simulink model "CASADI_MPC"  (R2023b)
settings: Solver=FixedStepAuto  StartTime=0.0  StopTime=15  FixedStep=0.002  RelTol=1e-3  EnableMultiTasking=on
undefined symbols (not defined in the file or in its folder): DiscIntNeverNeededParam
settings Model: ExtModeTrigDuration=10000  Creator=franc  LastModifiedBy=franc
settings SolverCC: AlgebraicLoopSolver=TrustRegion  PositivePriorityOrder=on
settings DataIOCC: ReturnWorkspaceOutputs=off
settings OptimizationCC: LifeSpan=inf
settings DebuggingCC: UnconnectedInputMsg=warning  UnconnectedOutputMsg=warning  UnconnectedLineMsg=warning  ArithmeticOperatorsInVariantConditions=warning
settings ModelReferenceCC: EnableRefExpFcnMdlSchedulingChecks=on
settings SFSimCC: SimUseLocalCustomCode=off  CustomCodeUndefinedFunction=UseInterfaceOnly
settings RTWCC: Description=QUARC Win64 Target  SystemTargetFile=quarc_win64.tlc  TemplateMakefile=quarc_default_tmf  RTWUseLocalCustomCode=off
settings CodeAppCC: StateflowObjectComments=on
settings STFCustomTargetCC: TargetPreCompLibLocation=C:\PROGRA~3\QUARC\lib\2016a\win64\release  ConcurrentExecutionCompliant=on  GRTInterface=on  SystemTargetFile=quarc_win64.tlc
settings GRTTargetCC: TargetPreCompLibLocation=C:\PROGRA~3\QUARC\lib\2016a\win64\release  ParMdlRefBuildCompliant=off  CompOptLevelCompliant=off  CombineOutputUpdateFcns=off  MatFileLogging=off  CPPClassGenCompliant=off  GRTInterface=on  UseToolchainInfoCompliant=off  ExtMode=on  ExtModeMexFile=quarc_comm
settings ConfigComp: CovMetricSettings=dswe

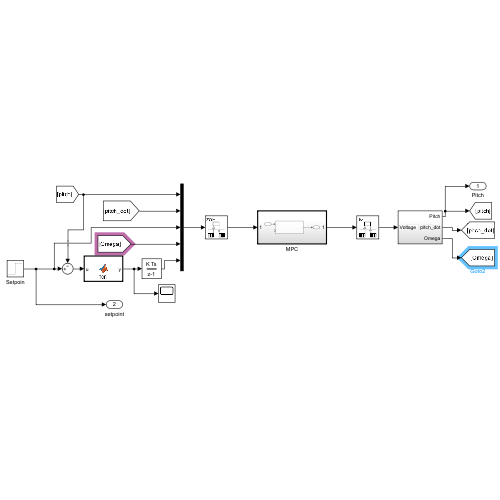
[thumbnail: Simulink's stored preview of the top-level diagram]
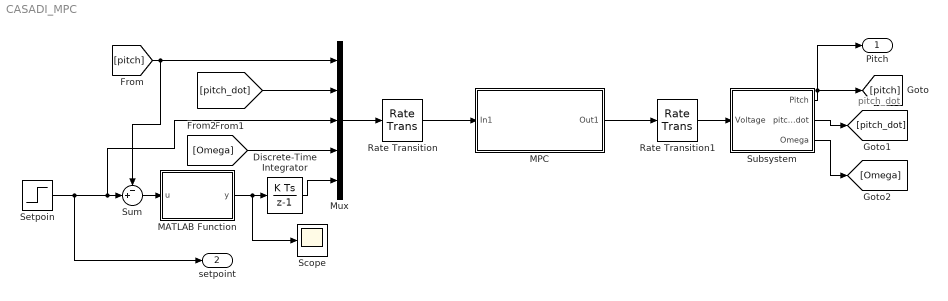
== system CASADI_MPC ==
  note: pitch_dot
  Discrete-Time Integrator : DiscreteIntegrator  SampleTime=-1  ICPrevOutput=DiscIntNeverNeededParam  ICPrevScaledInput=DiscIntNeverNeededParam
  MATLAB Function : MATLAB Function  TreatAsAtomicUnit=on
  MPC : Subsystem  TreatAsAtomicUnit=on  SystemSampleTime=0.1
  Mux : Mux  Inputs=5
  Rate Transition : RateTransition
  Rate Transition1 : RateTransition
  Scope : Scope
  Setpoin : Step  SampleTime=0
  Subsystem : Subsystem
  Sum : Sum  Inputs=-+|
  Pitch : Outport
  setpoint : Outport  Port=2
  wires:
  Setpoin/1 -> setpoint/1, Sum/2, Mux/3
  Rate Transition1/1 -> Subsystem/1(Voltage)
  Rate Transition/1 -> MPC/1(In1)
  Sum/1 -> MATLAB Function/1(u)
  Mux/1 -> Rate Transition/1
  Discrete-Time Integrator/1 -> Mux/5
  [Omega] -> Mux/4
  [pitch] -> Mux/1, Sum/1
  Subsystem/2(pitch_dot) -> [pitch_dot]
  [pitch_dot] -> Mux/2
  Subsystem/3(Omega) -> [Omega]
  Subsystem/1(Pitch) -> Pitch/1, [pitch]
  MPC/1(Out1) -> Rate Transition1/1
  MATLAB Function/1(y) -> Scope/1, Discrete-Time Integrator/1

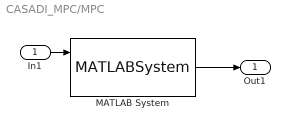
== system CASADI_MPC/MPC ==
  In1 : Inport
  MATLAB System : MATLABSystem  System=casadi_block  SimulateUsing=Interpreted execution
      mask Type: casadi_block
      mask Display:
      | disp('casadi_block');
      | port_label('input',1,'x');
      | port_label('input',2,'t');
      | port_label('output',1,'u');
  Out1 : Outport
  wires:
  In1/1 -> MATLAB System/1
  MATLAB System/1 -> Out1/1

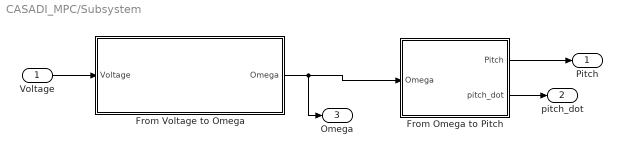
== system CASADI_MPC/Subsystem ==
  Voltage : Inport
  From Omega to Pitch : Subsystem
  From Voltage to Omega : Subsystem
  Pitch : Outport
  pitch_dot : Outport  Port=2
  Omega : Outport  Port=3
  wires:
  From Voltage to Omega/1(Omega) -> Omega/1, From Omega to Pitch/1(Omega)
  Voltage/1 -> From Voltage to Omega/1(Voltage)
  From Omega to Pitch/1(Pitch) -> Pitch/1
  From Omega to Pitch/2(pitch_dot) -> pitch_dot/1

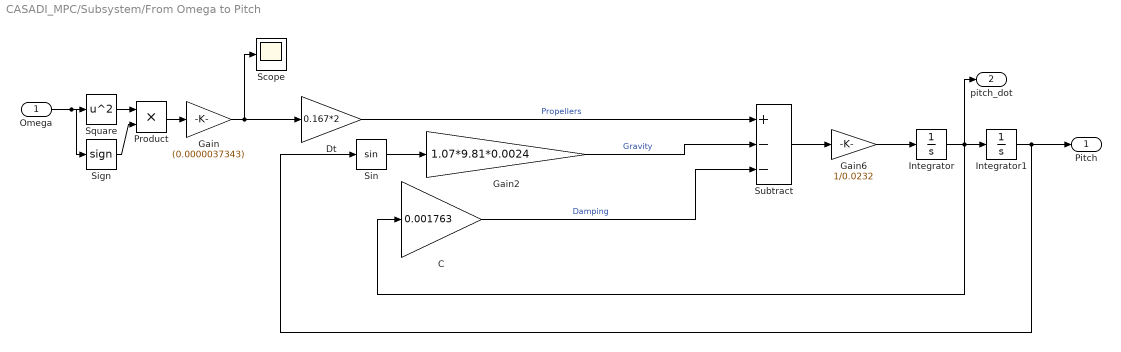
== system CASADI_MPC/Subsystem/From Omega to Pitch ==
  Omega : Inport
  C : Gain  Gain=0.001763
  Dt : Gain  Gain=0.167*2
  Gain : Gain  Gain=(0.0000037343)
  Gain2 : Gain  Gain=1.07*9.81*0.0024
  Gain6 : Gain  Gain=1/0.0232
  Integrator : Integrator
  Integrator1 : Integrator
  Product : Product
  Scope : Scope
  Sign : Signum  ZeroCross=off
  Sin : Trigonometry
  Square : Math  Operator=square
  Subtract : Sum  Inputs=+--
  Pitch : Outport
  pitch_dot : Outport  Port=2
  wires:
  Integrator1/1 -> Pitch/1, Sin/1
  Sin/1 -> Gain2/1
  Subtract/1 -> Gain6/1
  Gain2/1 -> Subtract/2  "Gravity"
  C/1 -> Subtract/3  "Damping"
  Omega/1 -> Sign/1, Square/1
  Gain6/1 -> Integrator/1
  Integrator/1 -> pitch_dot/1, Integrator1/1, C/1
  Dt/1 -> Subtract/1  "Propellers"
  Product/1 -> Gain/1
  Square/1 -> Product/1
  Sign/1 -> Product/2
  Gain/1 -> Scope/1, Dt/1

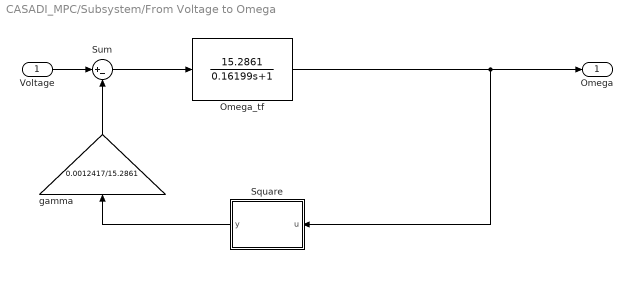
== system CASADI_MPC/Subsystem/From Voltage to Omega ==
  Voltage : Inport
  Omega_tf : TransferFcn  Numerator=15.2861  Denominator=[0.16199 1]
  Square : MATLAB Function  TreatAsAtomicUnit=on
  Sum : Sum  Inputs=|+-
  gamma : Gain  Gain=0.0012417/15.2861
  Omega : Outport
  wires:
  Voltage/1 -> Sum/1
  gamma/1 -> Sum/2
  Square/1(y) -> gamma/1
  Omega_tf/1 -> Omega/1, Square/1(u)
  Sum/1 -> Omega_tf/1

== matlab function CASADI_MPC/Subsystem/From Voltage to Omega/Square ==
  data: u input; y output
function y = fcn(u)
y=u^2*sign(u);

== matlab function CASADI_MPC/MATLAB Function ==
  data: u input; y output
function y = fcn(u)

y = max(min(u,1*pi/180),-1*pi/180);
